simulink model "quadrotorsim"  (Simulink 10.0)
settings: Solver=ode45  StartTime=0.0  StopTime=30  FixedStep=.01  RelTol=1e-3  EnableMultiTasking=on
undefined symbols (not defined in the file or in its folder): controller, P
libraries: simulink x1
settings Model: Creator=beard  LastModifiedBy=abara
settings DataIOCC: LimitDataPoints=on  SignalLoggingSaveFormat=ModelDataLogs  SignalLoggingName=sigsOut
settings OptimizationCC: BooleanDataType=off  InitFltsAndDblsToZero=on
settings DebuggingCC: SaveWithParameterizedLinksMsg=none  SignalResolutionControl=TryResolveAllWithWarning  MultiTaskDSMMsg=warning  MultiTaskCondExecSysMsg=none  FcnCallInpInsideContextMsg=warning  StateNameClashWarn=warning
settings HardwareCC: TargetBitPerPointer=64  TargetBitPerSizeT=64  TargetBitPerPtrDiffT=64  TargetLongLongMode=on  TargetIntDivRoundTo=Zero  TargetEndianess=LittleEndian  TargetWordSize=64  TargetHWDeviceType=MATLAB Host  ProdEqTarget=off
settings GRTTargetCC: TargetFcnLib=ansi_tfl_tmw.mat  ModelReferenceCompliant=off  GeneratePreprocessorConditionals=Disable all  MatFileLogging=off
settings ConfigComp: CovExternalEMLEnable=off

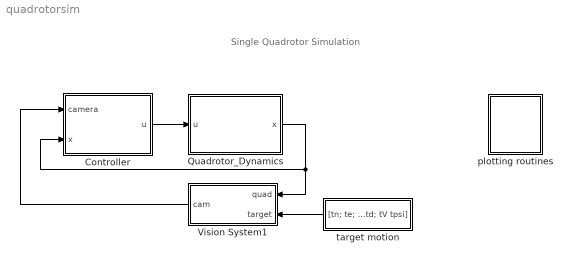
== system quadrotorsim ==
  note: Single Quadrotor Simulation
  Controller : Subsystem
  Quadrotor_Dynamics : Subsystem
  Vision System1 : Subsystem
  plotting routines : Subsystem
  target motion : Subsystem
  wires:
  Quadrotor_Dynamics/1(x) -> Vision System1/1(quad), Controller/2(x)
  Vision System1/1(cam) -> Controller/1(camera)
  target motion/1("[tn; te; td; tV tpsi]") -> Vision System1/2(target)
  Controller/1(u) -> Quadrotor_Dynamics/1(u)

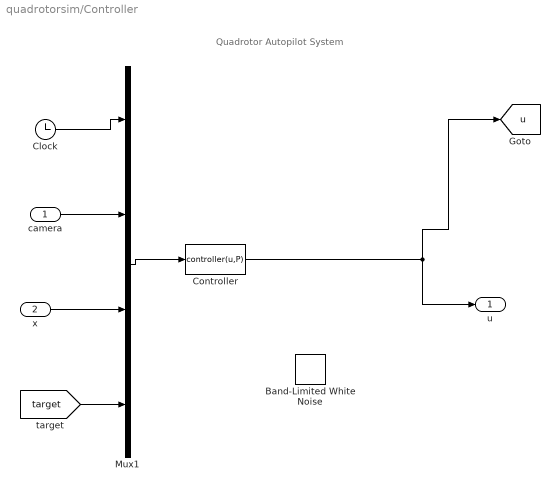
== system quadrotorsim/Controller ==
  note: Quadrotor Autopilot System
  camera : Inport
  x : Inport  Port=2
  Band-Limited White Noise : simulink/Sources/Band-Limited White Noise  Cov=[0.001]  Ts=0.03  seed=[10000]
  Clock : Clock
  Controller : MATLABFcn  MATLABFcn=controller(u,P)  OutputDimensions=4  SampleTime=P.Ts
  Mux1 : Mux
  u : Outport
  tag scope: u=global
  wires:
  Mux1/1 -> Controller/1
  camera/1 -> Mux1/2
  Clock/1 -> Mux1/1
  x/1 -> Mux1/3
  [target] -> Mux1/4
  Controller/1 -> [u], u/1

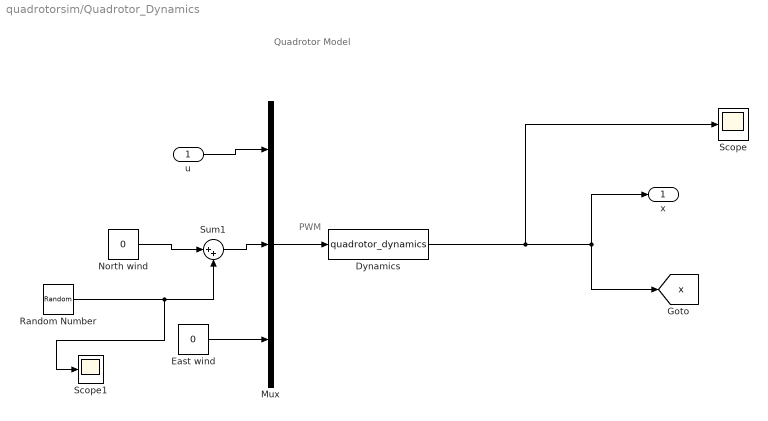
== system quadrotorsim/Quadrotor_Dynamics ==
  note: PWM
  note: Quadrotor Model
  u : Inport
  Dynamics : S-Function  FunctionName=quadrotor_dynamics  Parameters=P  SFunctionDeploymentMode=off  EnableBusSupport=off
  East wind : Constant  Value=0
  Mux : Mux  Inputs=3
  North wind : Constant  Value=0
  Random Number : RandomNumber  Seed=8  SampleTime=0.1
  Scope : Scope
  Scope1 : Scope
  Sum1 : Sum  Inputs=|++
  x : Outport
  tag scope: x=global
  wires:
  East wind/1 -> Mux/3
  Mux/1 -> Dynamics/1
  u/1 -> Mux/1
  North wind/1 -> Sum1/1
  Random Number/1 -> Scope1/1, Sum1/2
  Sum1/1 -> Mux/2
  Dynamics/1 -> Scope/1, [x], x/1

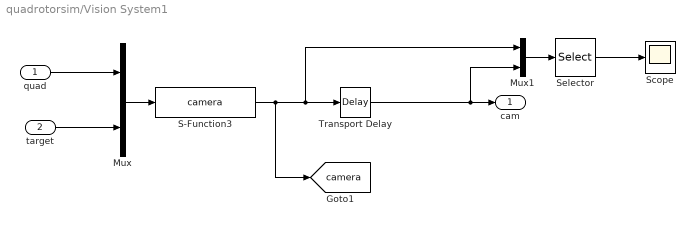
== system quadrotorsim/Vision System1 ==
  quad : Inport
  target : Inport  Port=2
  Mux : Mux  Inputs=2
  Mux1 : Mux  Inputs=2
  S-Function3 : S-Function  FunctionName=camera  Parameters=P  SFunctionDeploymentMode=off  EnableBusSupport=off
  Scope : Scope
  Selector : Selector  InputPortWidth=8  IndexOptions=Index vector (dialog)  Indices=[1 5]  OutputSizes=1
  Transport Delay : TransportDelay  DelayTime=P.Tcam
  cam : Outport
  tag scope: camera=global
  wires:
  target/1 -> Mux/2
  quad/1 -> Mux/1
  Mux/1 -> S-Function3/1
  S-Function3/1 -> [camera], Mux1/1, Transport Delay/1
  Mux1/1 -> Selector/1
  Selector/1 -> Scope/1
  Transport Delay/1 -> cam/1, Mux1/2

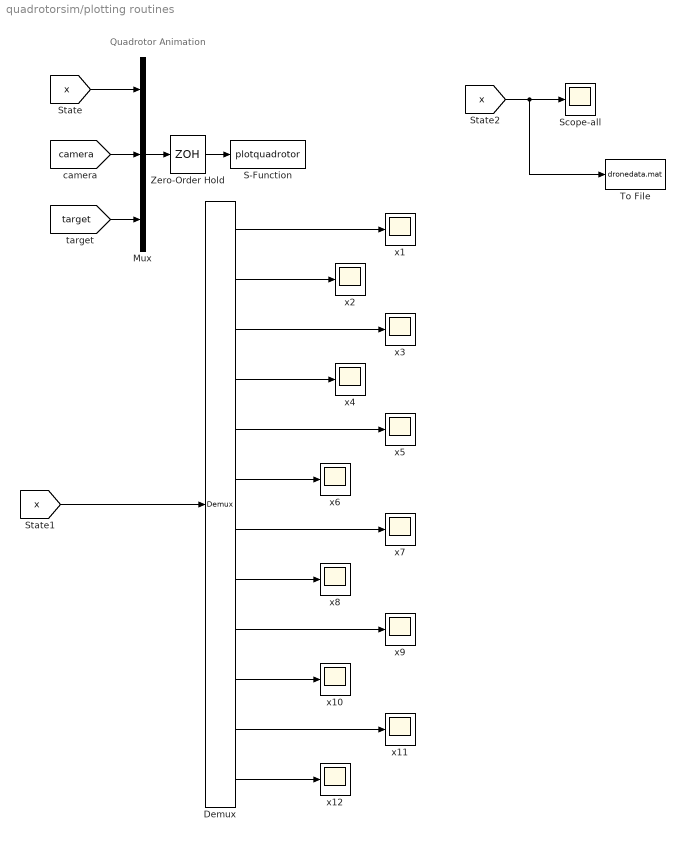
== system quadrotorsim/plotting routines ==
  note: Quadrotor Animation
  Demux : Demux  Outputs=12
  Mux : Mux  Inputs=3
  S-Function : S-Function  FunctionName=plotquadrotor  Parameters=P  SFunctionDeploymentMode=off  EnableBusSupport=off
  Scope-all : Scope
  To File : ToFile  Filename=dronedata.mat  SaveFormat=Timeseries
  Zero-Order Hold : ZeroOrderHold  SampleTime=2*P.Ts
  x{1..12} (12 alike) : Scope
  wires:
  [x] -> Mux/1
  Zero-Order Hold/1 -> S-Function/1
  Mux/1 -> Zero-Order Hold/1
  [target] -> Mux/3
  [camera] -> Mux/2
  [x] -> Demux/1
  Demux/1 -> x1/1
  Demux/2 -> x2/1
  Demux/3 -> x3/1
  Demux/4 -> x4/1
  Demux/5 -> x5/1
  Demux/6 -> x6/1
  Demux/7 -> x7/1
  Demux/8 -> x8/1
  Demux/9 -> x9/1
  Demux/10 -> x10/1
  Demux/11 -> x11/1
  Demux/12 -> x12/1
  [x] -> To File/1, Scope-all/1

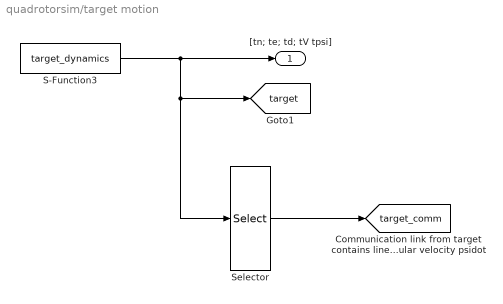
== system quadrotorsim/target motion ==
  S-Function3 : S-Function  FunctionName=target_dynamics  Parameters=P  SFunctionDeploymentMode=off  EnableBusSupport=off
  Selector : Selector  InputPortWidth=7  IndexOptions=Index vector (dialog)  Indices=[4, 6, 7]  OutputSizes=1
  "[tn; te; td; tV tpsi]" : Outport
  tag scope: target=global, target_comm=global
  wires:
  S-Function3/1 -> "[tn; te; td; tV tpsi]"/1, [target], Selector/1
  Selector/1 -> [target_comm]
